simulink model "SRF_PLL_test"  (R2025a)
settings: Solver=FixedStepAuto  StartTime=0.0  StopTime=0.2  FixedStep=1e-4  MinStep=0.0001  RelTol=1e-3
undefined symbols (not defined in the file): DiscIntNeverNeededParam
libraries: spsPLL3phLib x1, spsAlphaBetaZerotodq0Lib x1, slpidlib x1, spsabctoAlphaBetaZeroLib x1, spsdq0toabcLib x1
settings Model: Creator=li_hh  LastModifiedBy=li_hh
settings OptimizationCC: DefaultParameterBehavior=Inlined  EnhancedBackFolding=on  PassReuseOutputArgsAs=Individual arguments  ZeroExternalMemoryAtStartup=off  ZeroInternalMemoryAtStartup=off  OptimizeBlockOrder=speed  DifferentSizesBufferReuse=on  OptimizationCustomize=off  EfficientTunableParamExpr=on
settings DebuggingCC: ParameterTunabilityLossMsg=error
settings SFSimCC: MATLABDynamicMemAlloc=off
settings RTWCC: SystemTargetFile=ert.tlc  GenCodeOnly=on  TemplateMakefile=ert_default_tmf  Description=Embedded Coder
settings CodeAppCC: ForceParamTrailComments=on  IgnoreCustomStorageClasses=off  OperatorAnnotations=on  SimulinkDataObjDesc=on  SFDataObjDesc=on  InsertBlockDesc=on
settings ERTTargetCC: ExtModeTransport=0.0  ExtModeStaticAlloc=off  ExtModeMexFile=ext_comm  ExtModeIntrfLevel=Level1  ERTCustomFileTemplate=example_file_process.tlc  TargetLangStandard=C99 (ISO)  GenerateSampleERTMain=on  SupportContinuousTime=on

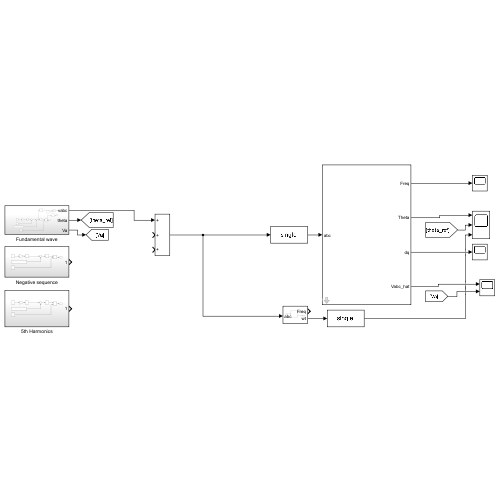
[thumbnail: Simulink's stored preview of the top-level diagram]
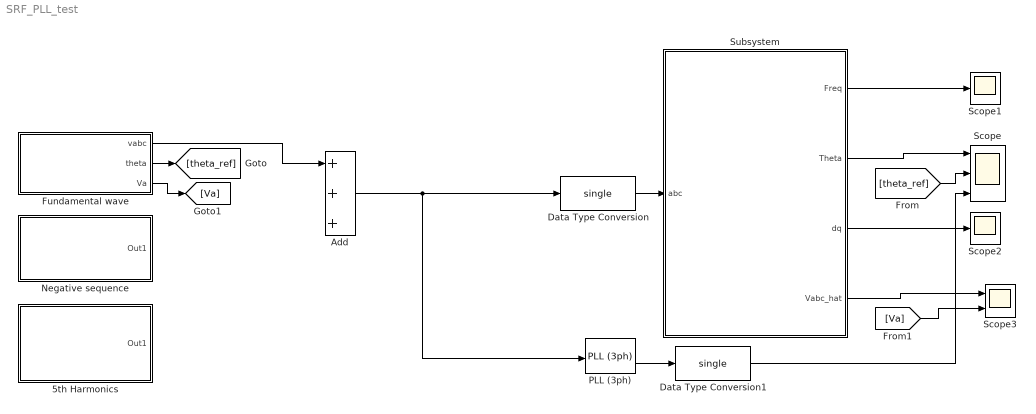
== system SRF_PLL_test ==
  5th Harmonics : Subsystem
  Add : Sum  Inputs=+++
  Data Type Conversion : DataTypeConversion  OutDataTypeStr=single  SaturateOnIntegerOverflow=off  RndMeth=Floor
  Data Type Conversion1 : DataTypeConversion  OutDataTypeStr=single  SaturateOnIntegerOverflow=off  RndMeth=Floor
  Fundamental wave : Subsystem
  Negative sequence : Subsystem
  PLL (3ph) : spsPLL3phLib/PLL (3ph)  Fmin=45  Par_Init=[0, 50]  ParK=[180, 3200, 1]  TcD=1e-4  MaxRateChangeFreq=12  FilterCutOffFreq=25  Ts=0  AGC=on
  Scope : Scope  NumInputPorts=3
      settings: ActiveDisplayYMinimum=-8.8264454256364484  ActiveDisplayYMaximum=11.020174998812013
  Scope1 : Scope
      settings: ActiveDisplayYMinimum=-1  ActiveDisplayYMaximum=1
  Scope2 : Scope
      settings: ActiveDisplayYMinimum=-548.01030731201172  ActiveDisplayYMaximum=549.778923034668  DataLoggingVariableName=ScopeData2
  Scope3 : Scope  NumInputPorts=2
      settings: ActiveDisplayYMinimum=-1997.6545600978561  ActiveDisplayYMaximum=1120.2605842812141  DataLoggingVariableName=ScopeData3
  Subsystem : Subsystem  mask{grid_freq_hz=50, damp=1/sqrt(2), omega_n=2*pi*30, Ts=0.0001}
      mask prompts: grid_freq_hz "Feedforward Grid Frequency (Hz)"; damp "Damping ratio"; omega_n "Natural frequency (rad/s)"; Ts "Sampling period(s)"
      mask DialogControl ParameterGroupVar Prompt: 参数
  wires:
  Subsystem/2(Theta) -> Scope/1
  [theta_ref] -> Scope/2
  Subsystem/1(Freq) -> Scope1/1
  Subsystem/3(dq) -> Scope2/1
  Subsystem/4(Vabc_hat) -> Scope3/1
  Data Type Conversion/1 -> Subsystem/1(abc)
  PLL (3ph)/2 -> Data Type Conversion1/1
  Add/1 -> PLL (3ph)/1, Data Type Conversion/1
  Fundamental wave/1(vabc) -> Add/1
  Fundamental wave/2(theta) -> [theta_ref]
  Fundamental wave/3(Va) -> [Va]
  Data Type Conversion1/1 -> Scope/3
  [Va] -> Scope3/2

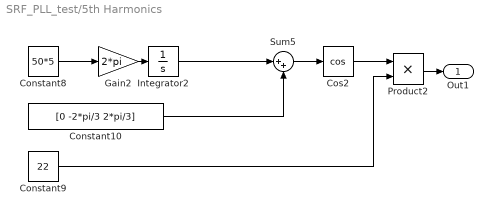
== system SRF_PLL_test/5th Harmonics ==
  Constant10 : Constant  Value=[0 -2*pi/3 2*pi/3]
  Constant8 : Constant  Value=50*5
  Constant9 : Constant  Value=22
  Cos2 : Trigonometry  Operator=cos
  Gain2 : Gain  Gain=2*pi
  Integrator2 : Integrator
  Product2 : Product
  Sum5 : Sum  Inputs=|++
  Out1 : Outport
  wires:
  Constant8/1 -> Gain2/1
  Constant9/1 -> Product2/2
  Cos2/1 -> Product2/1
  Product2/1 -> Out1/1
  Constant10/1 -> Sum5/2
  Integrator2/1 -> Sum5/1
  Gain2/1 -> Integrator2/1
  Sum5/1 -> Cos2/1

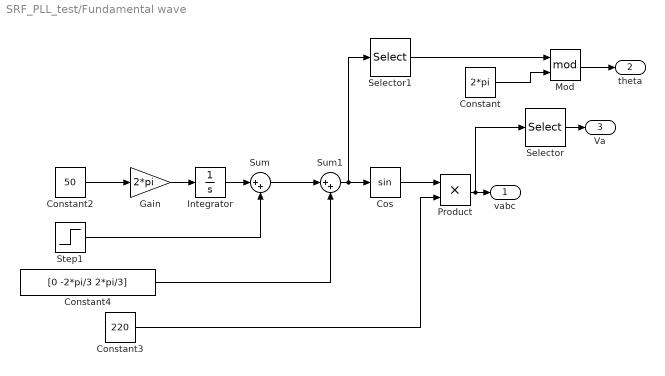
== system SRF_PLL_test/Fundamental wave ==
  Constant : Constant  Value=2*pi
  Constant2 : Constant  Value=50
  Constant3 : Constant  Value=220
  Constant4 : Constant  Value=[0 -2*pi/3 2*pi/3]
  Cos : Trigonometry
  Gain : Gain  Gain=2*pi
  Integrator : Integrator
  Mod : Math  Operator=mod
  Product : Product
  Selector : Selector  InputPortWidth=3  IndexOptions=Index vector (dialog)  Indices=[1]  OutputSizes=1
  Selector1 : Selector  InputPortWidth=3  IndexOptions=Index vector (dialog)  Indices=[1]  OutputSizes=1
  Step1 : Step  Time=0.1  After=-pi
  Sum : Sum  Inputs=|++
  Sum1 : Sum  Inputs=|++
  vabc : Outport
  theta : Outport  Port=2
  Va : Outport  Port=3
  wires:
  Step1/1 -> Sum/2
  Cos/1 -> Product/1
  Integrator/1 -> Sum/1
  Sum1/1 -> Selector1/1, Cos/1
  Constant3/1 -> Product/2
  Constant4/1 -> Sum1/2
  Sum/1 -> Sum1/1
  Constant2/1 -> Gain/1
  Product/1 -> Selector/1, vabc/1
  Gain/1 -> Integrator/1
  Selector/1 -> Va/1
  Mod/1 -> theta/1
  Constant/1 -> Mod/2
  Selector1/1 -> Mod/1

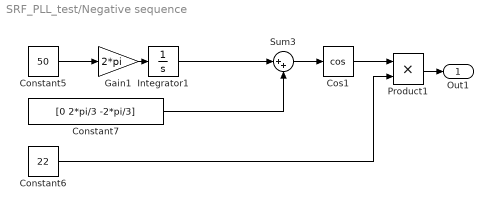
== system SRF_PLL_test/Negative sequence ==
  Constant5 : Constant  Value=50
  Constant6 : Constant  Value=22
  Constant7 : Constant  Value=[0 2*pi/3 -2*pi/3]
  Cos1 : Trigonometry  Operator=cos
  Gain1 : Gain  Gain=2*pi
  Integrator1 : Integrator
  Product1 : Product
  Sum3 : Sum  Inputs=|++
  Out1 : Outport
  wires:
  Integrator1/1 -> Sum3/1
  Cos1/1 -> Product1/1
  Constant7/1 -> Sum3/2
  Constant6/1 -> Product1/2
  Gain1/1 -> Integrator1/1
  Constant5/1 -> Gain1/1
  Product1/1 -> Out1/1
  Sum3/1 -> Cos1/1

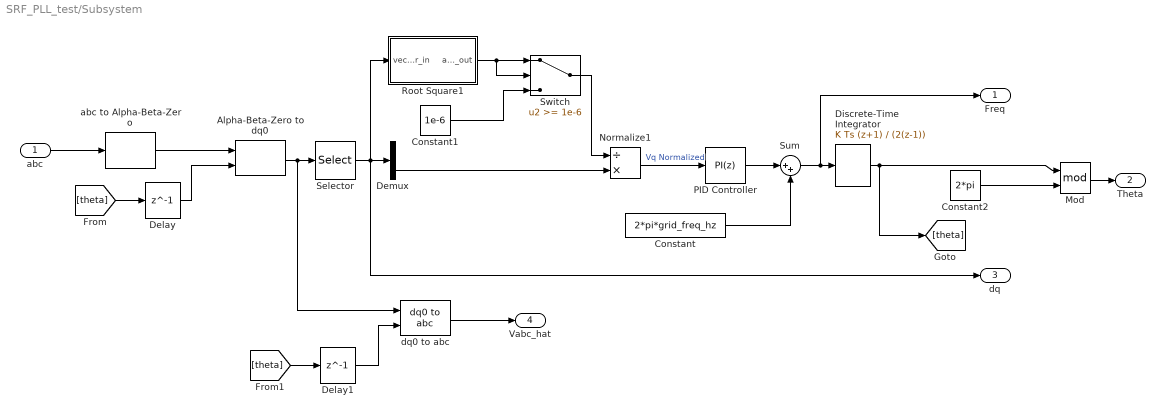
== system SRF_PLL_test/Subsystem ==
  abc : Inport
  Alpha-Beta-Zero to dq0 : spsAlphaBetaZerotodq0Lib/Alpha-Beta-Zero to dq0  Alignment=90 degrees behind phase A axis
  Constant : Constant  Value=2*pi*grid_freq_hz
  Constant1 : Constant  Value=1e-6
  Constant2 : Constant  Value=2*pi  OutDataTypeStr=single
  Delay : Delay  DelayLength=1  InputProcessing=Columns as channels (frame based)  SampleTime=Ts
  Delay1 : Delay  DelayLength=1  InputProcessing=Columns as channels (frame based)  SampleTime=Ts
  Demux : Demux  Outputs=2
  Discrete-Time Integrator : DiscreteIntegrator  IntegratorMethod=Integration: Trapezoidal  SampleTime=Ts  OutDataTypeStr=single  ICPrevOutput=DiscIntNeverNeededParam  ICPrevScaledInput=DiscIntNeverNeededParam
  Mod : Math  Operator=mod
  Normalize1 : Product  Inputs=/*
  PID Controller : slpidlib/PID Controller  Controller=PI  Form=Parallel  TimeDomain=Discrete-time  UseExternalTs=off  SampleTime=Ts  IntegratorMethod=Forward Euler  FilterMethod=Forward Euler  ControllerParametersSource=internal  P=2*damp*omega_n  I=omega_n*omega_n  UseKiTs=off  D=0  UseExternalDerivativeSource=off  N=100  UseFilter=on  TunerSelectOption=Transfer Function Based (PID Tuner App)  InitialConditionSource=internal  InitialConditionForIntegrator=0  InitialConditionForFilter=0  DifferentiatorICPrevScaledInput=0  ExternalReset=none  TrackingMode=off  Kt=1  LimitOutput=off  SatLimitsSource=internal  UpperSaturationLimit=inf  LowerSaturationLimit=-inf  LinearizeAsGain=on  AntiWindupMode=none  Kb=1  LimitIntegrator=off  UpperIntegratorSaturationLimit=inf  LowerIntegratorSaturationLimit=-inf  POutMin=[]  POutMax=[]  IOutMin=[]  IOutMax=[]  DOutMin=[]  DOutMax=[]  NOutMin=[]  NOutMax=[]  SumOutMin=[]  SumOutMax=[]  SaturationOutMin=[]  SaturationOutMax=[]  PParamMin=[]  PParamMax=[]  IParamMin=[]  IParamMax=[]  DParamMin=[]  DParamMax=[]  NParamMin=[]  NParamMax=[]  KbParamMin=[]  KbParamMax=[]  KtParamMin=[]  KtParamMax=[]  KbOutMin=[]  KbOutMax=[]  KtOutMin=[]  KtOutMax=[]  IntegratorOutMin=[]  IntegratorOutMax=[]  FilterOutMin=[]  FilterOutMax=[]  SumI1OutMin=[]  SumI1OutMax=[]  SumI2OutMin=[]  SumI2OutMax=[]  SumI3OutMin=[]  SumI3OutMax=[]  SumI4OutMin=[]  SumI4OutMax=[]  SumDOutMin=[]  SumDOutMax=[]  DifferentiatorOutMin=[]  DifferentiatorOutMax=[]  FilterDiffOutCoefMin=[]  FilterDiffOutCoefMax=[]  ReciprocalOutMin=[]  ReciprocalOutMax=[]  SumDenOutMin=[]  SumDenOutMax=[]  SumNumOutMin=[]  SumNumOutMax=[]  DivideOutMin=[]  DivideOutMax=[]  UdiffTsProdOutMin=[]  UdiffTsProdOutMax=[]  NTsProdOutMin=[]  NTsProdOutMax=[]  UintegralTsProdOutMin=[]  UintegralTsProdOutMax=[]  UngainTsProdOutMin=[]  UngainTsProdOutMax=[]  ClampingZeroOutDataTypeStr=Inherit: Inherit via back propagation  ClampingZeroOutMin=[]  ClampingZeroOutMax=[]  FilterDenConstantOutDataTypeStr=Inherit: Inherit via back propagation  FilterDenConstantOutMin=[]  FilterDenConstantOutMax=[]  PCopyOutDataTypeStr=Inherit: Inherit via back propagation  PCopyOutMin=[]  PCopyOutMax=[]  NCopyOutDataTypeStr=Inherit: Inherit via back propagation  NCopyOutMin=[]  NCopyOutMax=[]  IntegratorContinuousStateAttributes=''  IntegratorStateMustResolveToSignalObject=off  IntegratorRTWStateStorageClass=Auto  FilterContinuousStateAttributes=''  FilterStateMustResolveToSignalObject=off  FilterRTWStateStorageClass=Auto  ParallelPVariant=InternalParameters  IdealPVariant=Disabled  IVariant=InternalParameters  DVariant=Disabled  IntegratorVariant=Discrete  SatVariant=Disabled  AWVariant=Passthrough  PCopyVariant=Disabled  TRVariant=Disabled  FdbkBlocksVariant=Forward  IdealPFdbkVariant=Disabled  SatFdbkVariant=Disabled  DerivativeFilterVariant=Disabled  NVariant=Disabled  NCopyVariant=Disabled_SignalSpec  FilterICVariant=Disabled  IntegratorICVariant=InternalICs  ExternalResetVariant=Disabled  TRSumVariant=Passthrough  SumFdbkVariant=Disabled  SumVariant=Sum_PI  TsampFilterVariant=InternalTs  TsampNgainVariant=Passthrough  TsampIntegralVariant=Disabled_SignalSpec  ExternalSaturationOutDataTypeStr=Inherit: Same as second input  DerivativeSourceVariant=Disabled  PreIntVariant=InternalPreInt
  Root Square1 : Subsystem
  Selector : Selector  InputPortWidth=3  IndexOptions=Index vector (dialog)  Indices=[1 2]  OutputSizes=1
  Sum : Sum  Inputs=|++
  Switch : Switch  Threshold=1e-6  SaturateOnIntegerOverflow=off  InputSameDT=off
  abc to Alpha-Beta-Zero : spsabctoAlphaBetaZeroLib/abc to Alpha-Beta-Zero
  dq0 to abc : spsdq0toabcLib/dq0 to abc  Alignment=90 degrees behind phase A axis
  Freq : Outport
  Theta : Outport  Port=2
  dq : Outport  Port=3
  Vabc_hat : Outport  Port=4
  wires:
  Alpha-Beta-Zero to dq0/1 -> dq0 to abc/1, Selector/1
  PID Controller/1 -> Sum/1
  Normalize1/1 -> PID Controller/1  "Vq Normalized"
  Demux/2 -> Normalize1/2
  Sum/1 -> Discrete-Time Integrator/1, Freq/1
  Constant/1 -> Sum/2
  Discrete-Time Integrator/1 -> [theta], Mod/1
  abc/1 -> abc to Alpha-Beta-Zero/1
  abc to Alpha-Beta-Zero/1 -> Alpha-Beta-Zero to dq0/1
  [theta] -> Delay/1
  Root Square1/1(amp_out) -> Switch/2, Switch/1
  Switch/1 -> Normalize1/1
  Constant1/1 -> Switch/3
  Selector/1 -> dq/1, Root Square1/1(vector_in), Demux/1
  Delay/1 -> Alpha-Beta-Zero to dq0/2
  Mod/1 -> Theta/1
  Constant2/1 -> Mod/2
  [theta] -> Delay1/1
  Delay1/1 -> dq0 to abc/2
  dq0 to abc/1 -> Vabc_hat/1

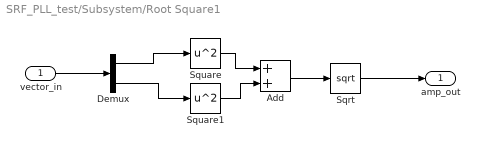
== system SRF_PLL_test/Subsystem/Root Square1 ==
  vector_in : Inport
  Add : Sum
  Demux : Demux  Outputs=2
  Sqrt : Sqrt
  Square : Math  Operator=square
  Square1 : Math  Operator=square
  amp_out : Outport
  wires:
  Square/1 -> Add/1
  Add/1 -> Sqrt/1
  Sqrt/1 -> amp_out/1
  Demux/2 -> Square1/1
  Square1/1 -> Add/2
  vector_in/1 -> Demux/1
  Demux/1 -> Square/1
